simulink model "ParentsApp"  (R2023b)
settings: Solver=FixedStepAuto  StartTime=0.0  StopTime=inf  RelTol=1e-3
libraries: androiduilib x7, androidcommunicationlib x7, androidaudiovideolib x3, simulink x2
settings Model: Creator=raj54  LastModifiedBy=Dell
settings OptimizationCC: EnhancedBackFolding=on  PassReuseOutputArgsThreshold=0  MaxStackSize=64  OptimizeBlockOrder=speed  DifferentSizesBufferReuse=on  OptimizationCustomize=off
settings DebuggingCC: ParameterTunabilityLossMsg=error
settings HardwareCC: ProdBitPerPointer=32  ProdBitPerSizeT=32  ProdBitPerPtrDiffT=32  ProdLargestAtomicInteger=Long  ProdLargestAtomicFloat=Double  ProdWordSize=32  ProdHWDeviceType=ARM Compatible->ARM Cortex  UseEmbeddedCoderFeatures=off  UseSimulinkCoderFeatures=off
settings ModelReferenceCC: EnableRefExpFcnMdlSchedulingChecks=on
settings SFSimCC: MATLABDynamicMemAlloc=off
settings RTWCC: Description=Embedded Coder  SystemTargetFile=ert.tlc  HardwareBoard=Android Device  TLCOptions="-aInlineSetEventsForThisBaseRateFcn=TLC_FALSE -aSuppressMultiTaskScheduler=TLC_FALSE  -aRateBasedStepFcn=0"  TemplateMakefile=ert_default_tmf  RTWVerbose=off  Toolchain=Android SDK/NDK Tools
settings CodeAppCC: ForceParamTrailComments=on  OperatorAnnotations=on
settings ERTTargetCC: ERTCustomFileBanners=off  SupportContinuousTime=on  SupportNonInlinedSFcns=on  RemoveResetFunc=off  ModelStepFunctionPrototypeControlCompliant=off

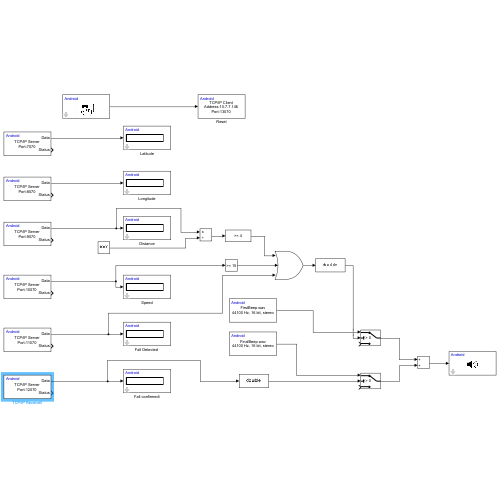
[thumbnail: Simulink's stored preview of the top-level diagram]
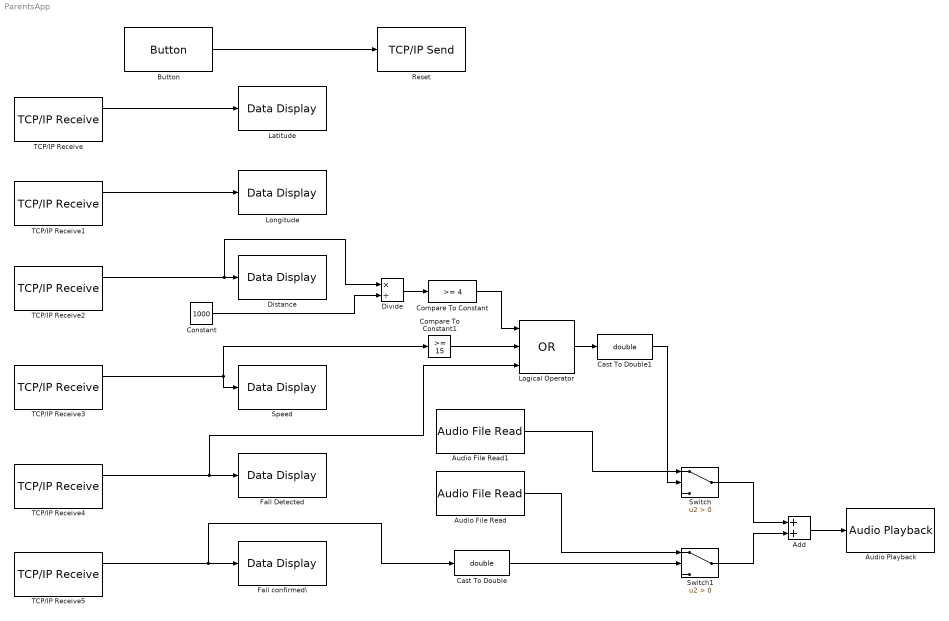
== system ParentsApp ==
  Add : Sum
  Audio File Read : androidaudiovideolib/Audio File Read  FileName=C:\Users\Dell\Downloads\FinalBeep.wav  FrameSize=4410
  Audio File Read1 : androidaudiovideolib/Audio File Read  FileName=C:\Users\Dell\Downloads\FirstBeep.wav  FrameSize=4410
  Audio Playback : androidaudiovideolib/Audio Playback  SampleFreq=44100  AudioSamplingFreq=44100  SampleTime=0.1  DeviceStr=0  QueueDuration=0  BlockPlatform=Android
  Button : androiduilib/Button  ButtonState=Not pressed  ButtonId=ParentsApp/Button  State=off  SampleTime=0.1  BlockPlatform=Android
  Cast To Double : DataTypeConversion  OutDataTypeStr=double  SaturateOnIntegerOverflow=off  RndMeth=Floor
  Cast To Double1 : DataTypeConversion  OutDataTypeStr=double  SaturateOnIntegerOverflow=off  RndMeth=Floor
  Compare To Constant : simulink/Logic and Bit Operations/Compare To Constant  relop=>=  const=4  OutDataTypeStr=boolean
  Compare To Constant1 : simulink/Logic and Bit Operations/Compare To Constant  relop=>=  const=15  OutDataTypeStr=boolean
  Constant : Constant  Value=1000
  Distance : androiduilib/Data Display  DataDisplayId=ParentsApp/Distance  Format=Float  Precision=6  SimulateUsing=Code generation  blockPlatform=Android
  Divide : Product  Inputs=*/
  "Fall Detected " : androiduilib/Data Display  DataDisplayId=ParentsApp/Fall_Detected_  Format=Float  Precision=6  SimulateUsing=Code generation  blockPlatform=Android
  Fall confirmed\ : androiduilib/Data Display  DataDisplayId=ParentsApp/Fall_confirmed\  Format=Float  Precision=6  SimulateUsing=Code generation  blockPlatform=Android
  Latitude : androiduilib/Data Display  DataDisplayId=ParentsApp/Latitude  Format=Float  Precision=6  SimulateUsing=Code generation  blockPlatform=Android
  Logical Operator : Logic  Operator=OR  Inputs=3  IconShape=distinctive  AllPortsSameDT=off  OutDataTypeStr=boolean
  Longitude : androiduilib/Data Display  DataDisplayId=ParentsApp/Longitude  Format=Float  Precision=6  SimulateUsing=Code generation  blockPlatform=Android
  Reset : androidcommunicationlib/TCP//IP Send  TCPSendId=ParentsApp/Reset  Mode_=Client  LocalServerPort_=25000  RemoteAddr_=10.7.7.146  RemoteServerPort_=13070  ClientPortBindingSelection_=off  ClientPortToBind_=35000  BlockingMode_=off  BlockTimeout_=0.1
  Speed : androiduilib/Data Display  DataDisplayId=ParentsApp/Speed  Format=Float  Precision=6  SimulateUsing=Code generation  blockPlatform=Android
  Switch : Switch  Criteria=u2 > Threshold  SaturateOnIntegerOverflow=off  InputSameDT=off
  Switch1 : Switch  Criteria=u2 > Threshold  SaturateOnIntegerOverflow=off  InputSameDT=off
  TCP/IP Receive : androidcommunicationlib/TCP//IP Receive  TCPReceiveId=ParentsApp/TCP//IP_Receive  Mode_=Server  LocalServerPort_=7070  RemoteAddr_=127.0.0.1  RemoteServerPort_=25000  DataType_=uint8  DataSize_=1  SampleTime_=4  ClientPortBindingSelection_=off  ClientPortToBind_=35000  BlockingMode_=on  BlockTimeout_=4.1
  TCP/IP Receive1 : androidcommunicationlib/TCP//IP Receive  TCPReceiveId=ParentsApp/TCP//IP_Receive1  Mode_=Server  LocalServerPort_=8070  RemoteAddr_=127.0.0.1  RemoteServerPort_=25000  DataType_=uint8  DataSize_=1  SampleTime_=4  ClientPortBindingSelection_=off  ClientPortToBind_=35000  BlockingMode_=on  BlockTimeout_=4.1
  TCP/IP Receive2 : androidcommunicationlib/TCP//IP Receive  TCPReceiveId=ParentsApp/TCP//IP_Receive2  Mode_=Server  LocalServerPort_=9070  RemoteAddr_=127.0.0.1  RemoteServerPort_=25000  DataType_=uint8  DataSize_=1  SampleTime_=4  ClientPortBindingSelection_=off  ClientPortToBind_=35000  BlockingMode_=on  BlockTimeout_=4.1
  TCP/IP Receive3 : androidcommunicationlib/TCP//IP Receive  TCPReceiveId=ParentsApp/TCP//IP_Receive3  Mode_=Server  LocalServerPort_=10070  RemoteAddr_=127.0.0.1  RemoteServerPort_=25000  DataType_=uint8  DataSize_=1  SampleTime_=4  ClientPortBindingSelection_=off  ClientPortToBind_=35000  BlockingMode_=on  BlockTimeout_=4.1
  TCP/IP Receive4 : androidcommunicationlib/TCP//IP Receive  TCPReceiveId=ParentsApp/TCP//IP_Receive4  Mode_=Server  LocalServerPort_=11070  RemoteAddr_=127.0.0.1  RemoteServerPort_=25000  DataType_=boolean  DataSize_=1  SampleTime_=4  ClientPortBindingSelection_=off  ClientPortToBind_=35000  BlockingMode_=on  BlockTimeout_=4.1
  TCP/IP Receive5 : androidcommunicationlib/TCP//IP Receive  TCPReceiveId=ParentsApp/TCP//IP_Receive5  Mode_=Server  LocalServerPort_=12070  RemoteAddr_=127.0.0.1  RemoteServerPort_=25000  DataType_=boolean  DataSize_=1  SampleTime_=4  ClientPortBindingSelection_=off  ClientPortToBind_=35000  BlockingMode_=on  BlockTimeout_=4.1
  wires:
  TCP/IP Receive/1 -> Latitude/1
  TCP/IP Receive1/1 -> Longitude/1
  TCP/IP Receive2/1 -> Divide/1, Distance/1
  TCP/IP Receive3/1 -> Speed/1, Compare To Constant1/1
  TCP/IP Receive4/1 -> Logical Operator/3, "Fall Detected "/1
  TCP/IP Receive5/1 -> Cast To Double/1, Fall confirmed\/1
  Compare To Constant/1 -> Logical Operator/1
  Compare To Constant1/1 -> Logical Operator/2
  Constant/1 -> Divide/2
  Divide/1 -> Compare To Constant/1
  Button/1 -> Reset/1
  Logical Operator/1 -> Cast To Double1/1
  Cast To Double1/1 -> Switch/2
  Cast To Double/1 -> Switch1/2
  Audio File Read/1 -> Switch1/1
  Audio File Read1/1 -> Switch/1
  Switch/1 -> Add/1
  Switch1/1 -> Add/2
  Add/1 -> Audio Playback/1
